simulink model "SIL_TMS"  (R2023b)
settings: Solver=VariableStepAuto  StartTime=0.0  StopTime=10.0  RelTol=1e-3
settings Model: Creator=schro  LastModifiedBy=schro
settings DataIOCC: ExternalInput=temp.getElement('Temp')  LoadExternalInput=on  OutputSaveName=MIL_out  LoggingToFile=on  LoggingFileName=MIL_out.mat
settings OptimizationCC: DefaultParameterBehavior=Inlined  EnhancedBackFolding=on  PassReuseOutputArgsAs=Individual arguments  ZeroExternalMemoryAtStartup=off  ZeroInternalMemoryAtStartup=off  OptimizeBlockOrder=speed  DifferentSizesBufferReuse=on  OptimizationCustomize=off  EfficientTunableParamExpr=on
settings DebuggingCC: ParameterTunabilityLossMsg=error
settings HardwareCC: ProdBitPerPointer=32  ProdBitPerSizeT=32  ProdBitPerPtrDiffT=32  ProdLargestAtomicFloat=None  ProdWordSize=32  ProdHWDeviceType=Atmel->AVR (32-bit)
settings ModelReferenceCC: EnableRefExpFcnMdlSchedulingChecks=on
settings SFSimCC: MATLABDynamicMemAlloc=off
settings RTWCC: Description=Embedded Coder  SystemTargetFile=ert.tlc  TemplateMakefile=ert_default_tmf
settings CodeAppCC: ForceParamTrailComments=on  IgnoreCustomStorageClasses=off  OperatorAnnotations=on  SimulinkDataObjDesc=on  SFDataObjDesc=on  InsertBlockDesc=on
settings ERTTargetCC: TargetLangStandard=C99 (ISO)  GenerateSampleERTMain=on  InlinedParameterPlacement=NonHierarchical  ERTCustomFileTemplate=example_file_process.tlc
settings ConfigComp: DVTestSuiteOptimization=Auto  DVDetectOutOfBounds=on  DVModelReferenceHarness=on  DVHarnessSource=Signal Editor  DVRebuildModelRepresentation=IfChangeIsDetected

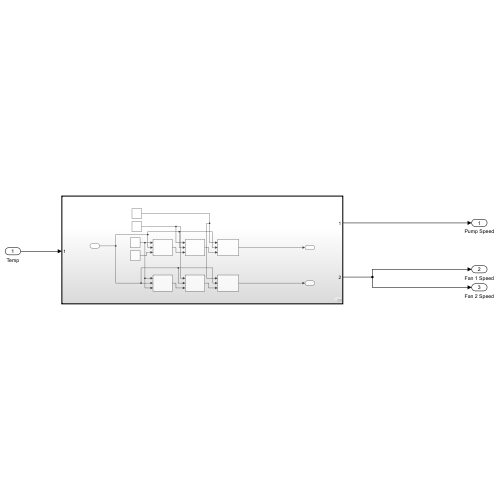
[thumbnail: Simulink's stored preview of the top-level diagram]
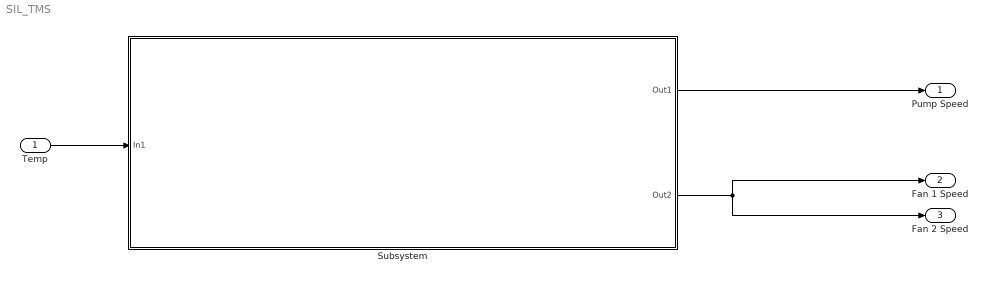
== system SIL_TMS ==
  Temp : Inport
  Subsystem : Subsystem  TreatAsAtomicUnit=on
  Pump Speed : Outport
  Fan 1 Speed : Outport  Port=2
  Fan 2 Speed : Outport  Port=3
  wires:
  Subsystem/2(Out2) -> Fan 1 Speed/1, Fan 2 Speed/1
  Temp/1 -> Subsystem/1(In1)
  Subsystem/1(Out1) -> Pump Speed/1

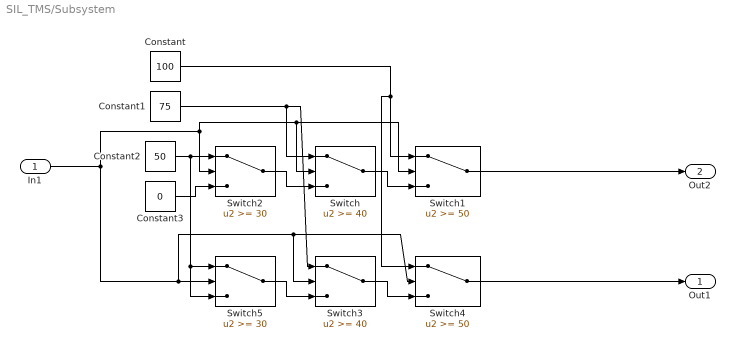
== system SIL_TMS/Subsystem ==
  In1 : Inport
  Constant : Constant  Value=100
  Constant1 : Constant  Value=75
  Constant2 : Constant  Value=50
  Constant3 : Constant  Value=0
  Switch : Switch  Threshold=40  SaturateOnIntegerOverflow=off  InputSameDT=off
  Switch1 : Switch  Threshold=50  SaturateOnIntegerOverflow=off  InputSameDT=off
  Switch2 : Switch  Threshold=30  SaturateOnIntegerOverflow=off  InputSameDT=off
  Switch3 : Switch  Threshold=40  SaturateOnIntegerOverflow=off  InputSameDT=off
  Switch4 : Switch  Threshold=50  SaturateOnIntegerOverflow=off  InputSameDT=off
  Switch5 : Switch  Threshold=30  SaturateOnIntegerOverflow=off  InputSameDT=off
  Out1 : Outport
  Out2 : Outport  Port=2
  wires:
  Constant2/1 -> Switch5/3, Switch5/1, Switch2/1
  Switch1/1 -> Out2/1
  Switch3/1 -> Switch4/3
  Switch5/1 -> Switch3/3
  Constant1/1 -> Switch3/1, Switch/1
  Constant/1 -> Switch4/1, Switch1/1
  Switch/1 -> Switch1/3
  Switch2/1 -> Switch/3
  Constant3/1 -> Switch2/3
  In1/1 -> Switch4/2, Switch3/2, Switch5/2, Switch/2, Switch1/2, Switch2/2
  Switch4/1 -> Out1/1
